simulink model "PILS"  (R2023a)
settings: Solver=daessc  StartTime=0.0  StopTime=1800  MaxStep=0.1  RelTol=1e-3
values from neighbouring files (symbols this model uses):
  Max_Power = 100000    [setHESSParam.m]    (also in setHESSParamv2.m)
  sim_case = i    [create_SOC_dataset.m]    (also in create_csv.m = 2; setHESSParam.m = 6; setHESSParamv2.m = 6)
undefined symbols (not defined in the file or in its folder): Battery, Capacitor, Ri
libraries: fl_lib x41, nesl_utility x22, dspstat3 x4, rllib x3, batteryecm_lib x1, autolibshared x1
(part 2 of 2)

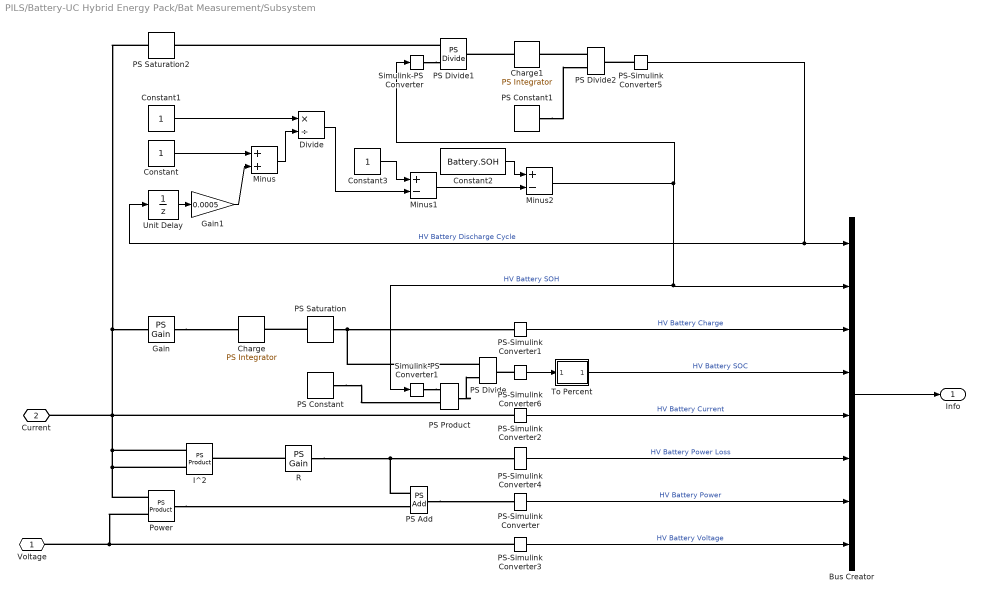
== system PILS/Battery-UC Hybrid Energy Pack/Bat Measurement/Subsystem ==
  Bus Creator : BusCreator  Inputs=8
  Charge : fl_lib/Physical Signals/Linear Operators/PS Integrator  reset_method=foundation.enum.IntegratorResetSpec.None  initial_condition_spec=foundation.enum.IntegratorICSpec.Internal  saturation_spec=foundation.enum.IntegratorSaturationSpec.None  saturation_source_spec=foundation.enum.IntegratorSaturationSourceSpec.Internal  x0=Battery.InitialCharge A*hr  xu=inf s  xl=-inf s
      settings: AttributesFormatString=%<x0> [%<x0_unit>]
  Charge1 : fl_lib/Physical Signals/Linear Operators/PS Integrator  reset_method=foundation.enum.IntegratorResetSpec.None  initial_condition_spec=foundation.enum.IntegratorICSpec.Internal  saturation_spec=foundation.enum.IntegratorSaturationSpec.None  saturation_source_spec=foundation.enum.IntegratorSaturationSourceSpec.Internal  x0=0 A*hr  xu=inf s  xl=-inf s
      settings: AttributesFormatString=%<x0> [%<x0_unit>]
  Constant : Constant
  Constant1 : Constant
  Constant2 : Constant  Value=Battery.SOH
  Constant3 : Constant
  Divide : Product  Inputs=*/
  Gain : fl_lib/Physical Signals/Functions/PS Gain  gain=-1
      settings: AttributesFormatString=%<gain>
  Gain1 : Gain  Gain=0.0005
  I^2 : fl_lib/Physical Signals/Functions/PS Product
  Minus : Sum
  Minus1 : Sum  Inputs=+-
  Minus2 : Sum  Inputs=+-
  PS Add : fl_lib/Physical Signals/Functions/PS Add
  PS Constant : fl_lib/Physical Signals/Sources/PS Constant  constant=Battery.Capacity A*hr
      settings: AttributesFormatString=%<constant> [%<constant_unit>]
  PS Constant1 : fl_lib/Physical Signals/Sources/PS Constant  constant=Battery.Capacity A*hr
  PS Divide : fl_lib/Physical Signals/Functions/PS Divide
  PS Divide1 : fl_lib/Physical Signals/Functions/PS Divide
  PS Divide2 : fl_lib/Physical Signals/Functions/PS Divide
  PS Product : fl_lib/Physical Signals/Functions/PS Product
  PS Saturation : fl_lib/Physical Signals/Nonlinear Operators/PS Saturation  upper_limit=Battery.Capacity A*hr  lower_limit=0 A*hr
      settings: AttributesFormatString=|
      | Upper: %<upper_limit>
      | Lower: %<lower_limit>
  PS Saturation2 : fl_lib/Physical Signals/Nonlinear Operators/PS Saturation  upper_limit=500 A  lower_limit=0 A
  PS-Simulink Converter : nesl_utility/PS-Simulink Converter  PhysicalDomain=network_engine_domain  SubClassName=ps_output  LeftPortType=input  RightPortType=output  PseudoPeriodic=off  Frequencies=[]  VectorFormat=1-D array  Unit=W  AffineConversion=off
  PS-Simulink Converter1 : nesl_utility/PS-Simulink Converter  PhysicalDomain=network_engine_domain  SubClassName=ps_output  LeftPortType=input  RightPortType=output  PseudoPeriodic=off  Frequencies=[]  VectorFormat=1-D array  Unit=A*hr  AffineConversion=off
  PS-Simulink Converter2 : nesl_utility/PS-Simulink Converter  PhysicalDomain=network_engine_domain  SubClassName=ps_output  LeftPortType=input  RightPortType=output  PseudoPeriodic=off  Frequencies=[]  VectorFormat=1-D array  Unit=A  AffineConversion=off
  PS-Simulink Converter3 : nesl_utility/PS-Simulink Converter  PhysicalDomain=network_engine_domain  SubClassName=ps_output  LeftPortType=input  RightPortType=output  PseudoPeriodic=off  Frequencies=[]  VectorFormat=1-D array  Unit=V  AffineConversion=off
  PS-Simulink Converter4 : nesl_utility/PS-Simulink Converter  PhysicalDomain=network_engine_domain  SubClassName=ps_output  LeftPortType=input  RightPortType=output  PseudoPeriodic=off  Frequencies=[]  VectorFormat=1-D array  Unit=W  AffineConversion=off
  PS-Simulink Converter5 : nesl_utility/PS-Simulink Converter  PhysicalDomain=network_engine_domain  SubClassName=ps_output  LeftPortType=input  RightPortType=output  PseudoPeriodic=off  Frequencies=[]  VectorFormat=inherit  Unit=1  AffineConversion=off
  PS-Simulink Converter6 : nesl_utility/PS-Simulink Converter  PhysicalDomain=network_engine_domain  SubClassName=ps_output  LeftPortType=input  RightPortType=output  PseudoPeriodic=off  Frequencies=[]  VectorFormat=1-D array  Unit=1  AffineConversion=off
  Power : fl_lib/Physical Signals/Functions/PS Product
  R : fl_lib/Physical Signals/Functions/PS Gain  gain=Battery.InternalResistance Ohm
      settings: AttributesFormatString=%<gain> [%<gain_unit>]
  Simulink-PS Converter : nesl_utility/Simulink-PS Converter  PhysicalDomain=network_engine_domain  SubClassName=ps_input  LeftPortType=input  RightPortType=output  PseudoPeriodic=off  Frequencies=[]  NoiseDistribution=none  NoiseParameters=[]  Unit=1  AffineConversion=off  FilteringAndDerivatives=provide  SimscapeFilterOrder=1  InputFilterTimeConstant=0.001  UdotUserProvided=0
  Simulink-PS Converter1 : nesl_utility/Simulink-PS Converter  PhysicalDomain=network_engine_domain  SubClassName=ps_input  LeftPortType=input  RightPortType=output  PseudoPeriodic=off  Frequencies=[]  NoiseDistribution=none  NoiseParameters=[]  Unit=1  AffineConversion=off  FilteringAndDerivatives=provide  SimscapeFilterOrder=1  InputFilterTimeConstant=0.001  UdotUserProvided=0
  To Percent : Subsystem
  Unit Delay : UnitDelay  SampleTime=-1  HasFrameUpgradeWarning=on
  Voltage : PMIOPort  Side=Left
  Current : PMIOPort  Port=2  Side=Left
  Info : Outport
  wires:
  PS-Simulink Converter4/1 -> Bus Creator/6  "HV Battery Power Loss"
  PS-Simulink Converter3/1 -> Bus Creator/8  "HV Battery Voltage"
  PS-Simulink Converter1/1 -> Bus Creator/3  "HV Battery Charge"
  Bus Creator/1 -> Info/1
  To Percent/1(Out1) -> Bus Creator/4  "HV Battery SOC"
  PS-Simulink Converter/1 -> Bus Creator/7  "HV Battery Power"
  PS-Simulink Converter6/1 -> To Percent/1(In1)
  PS-Simulink Converter2/1 -> Bus Creator/5  "HV Battery Current"
  Constant/1 -> Minus/1
  Gain1/1 -> Minus/2
  Unit Delay/1 -> Gain1/1
  Divide/1 -> Minus1/2
  Constant1/1 -> Divide/1
  Minus/1 -> Divide/2
  PS-Simulink Converter5/1 -> Bus Creator/1, Unit Delay/1  "HV Battery Discharge Cycle"
  Constant3/1 -> Minus1/1
  Constant2/1 -> Minus2/1
  Minus1/1 -> Minus2/2
  Minus2/1 -> Simulink-PS Converter1/1, Bus Creator/2, Simulink-PS Converter/1  "HV Battery SOH"
  connections:
  PS Divide/LConn1 -- PS-Simulink Converter1/LConn1 -- PS Saturation/RConn1
  Power/LConn1 -- Voltage/RConn1 -- PS-Simulink Converter3/LConn1
  R/RConn1 -- PS Add/LConn1 -- PS-Simulink Converter4/LConn1
  Power/LConn2 -- I^2/LConn1 -- Current/RConn1 -- PS Saturation2/LConn1 -- Gain/LConn1 -- PS-Simulink Converter2/LConn1 -- I^2/LConn2
  PS Add/RConn1 -- PS-Simulink Converter/LConn1
  R/LConn1 -- I^2/RConn1
  PS Saturation/LConn1 -- Charge/RConn1
  Gain/RConn1 -- Charge/LConn1
  PS-Simulink Converter6/LConn1 -- PS Divide/RConn1
  Power/RConn1 -- PS Add/LConn2
  PS Divide1/LConn1 -- PS Saturation2/RConn1
  Charge1/LConn1 -- PS Divide1/RConn1
  PS Divide2/LConn1 -- Charge1/RConn1
  PS Constant1/RConn1 -- PS Divide2/LConn2
  PS-Simulink Converter5/LConn1 -- PS Divide2/RConn1
  Simulink-PS Converter/RConn1 -- PS Divide1/LConn2
  PS Product/RConn1 -- PS Divide/LConn2
  PS Constant/RConn1 -- PS Product/LConn2
  Simulink-PS Converter1/RConn1 -- PS Product/LConn1

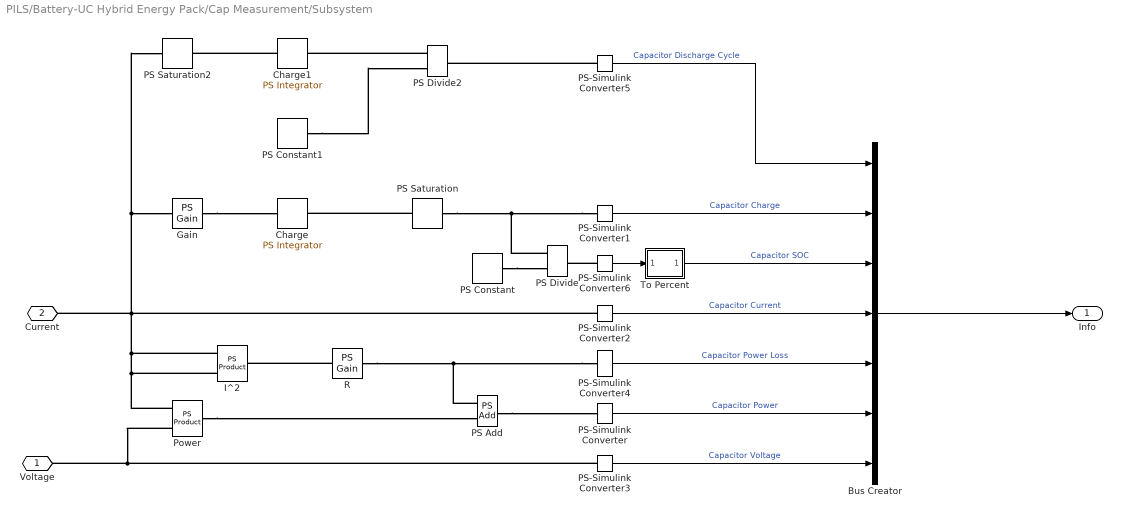
== system PILS/Battery-UC Hybrid Energy Pack/Cap Measurement/Subsystem ==
  Bus Creator : BusCreator  Inputs=7
  Charge : fl_lib/Physical Signals/Linear Operators/PS Integrator  reset_method=foundation.enum.IntegratorResetSpec.None  initial_condition_spec=foundation.enum.IntegratorICSpec.Internal  saturation_spec=foundation.enum.IntegratorSaturationSpec.None  saturation_source_spec=foundation.enum.IntegratorSaturationSourceSpec.Internal  x0=Capacitor.Capacity A*hr  xu=inf s  xl=-inf s
      settings: AttributesFormatString=%<x0> [%<x0_unit>]
  Charge1 : fl_lib/Physical Signals/Linear Operators/PS Integrator  reset_method=foundation.enum.IntegratorResetSpec.None  initial_condition_spec=foundation.enum.IntegratorICSpec.Internal  saturation_spec=foundation.enum.IntegratorSaturationSpec.None  saturation_source_spec=foundation.enum.IntegratorSaturationSourceSpec.Internal  x0=0 A*hr  xu=inf s  xl=-inf s
      settings: AttributesFormatString=%<x0> [%<x0_unit>]
  Gain : fl_lib/Physical Signals/Functions/PS Gain  gain=-1
      settings: AttributesFormatString=%<gain>
  I^2 : fl_lib/Physical Signals/Functions/PS Product
  PS Add : fl_lib/Physical Signals/Functions/PS Add
  PS Constant : fl_lib/Physical Signals/Sources/PS Constant  constant=Capacitor.Capacity A*hr
      settings: AttributesFormatString=%<constant> [%<constant_unit>]
  PS Constant1 : fl_lib/Physical Signals/Sources/PS Constant  constant=Capacitor.Capacity A*hr
      settings: AttributesFormatString=%<constant> [%<constant_unit>]
  PS Divide : fl_lib/Physical Signals/Functions/PS Divide
  PS Divide2 : fl_lib/Physical Signals/Functions/PS Divide
  PS Saturation : fl_lib/Physical Signals/Nonlinear Operators/PS Saturation  upper_limit=Capacitor.Capacity A*hr  lower_limit=0 A*hr
      settings: AttributesFormatString=|
      | Upper: %<upper_limit>
      | Lower: %<lower_limit>
  PS Saturation2 : fl_lib/Physical Signals/Nonlinear Operators/PS Saturation  upper_limit=500 A  lower_limit=0 A
  PS-Simulink Converter : nesl_utility/PS-Simulink Converter  PhysicalDomain=network_engine_domain  SubClassName=ps_output  LeftPortType=input  RightPortType=output  PseudoPeriodic=off  Frequencies=[]  VectorFormat=1-D array  Unit=W  AffineConversion=off
  PS-Simulink Converter1 : nesl_utility/PS-Simulink Converter  PhysicalDomain=network_engine_domain  SubClassName=ps_output  LeftPortType=input  RightPortType=output  PseudoPeriodic=off  Frequencies=[]  VectorFormat=1-D array  Unit=A*hr  AffineConversion=off
  PS-Simulink Converter2 : nesl_utility/PS-Simulink Converter  PhysicalDomain=network_engine_domain  SubClassName=ps_output  LeftPortType=input  RightPortType=output  PseudoPeriodic=off  Frequencies=[]  VectorFormat=1-D array  Unit=A  AffineConversion=off
  PS-Simulink Converter3 : nesl_utility/PS-Simulink Converter  PhysicalDomain=network_engine_domain  SubClassName=ps_output  LeftPortType=input  RightPortType=output  PseudoPeriodic=off  Frequencies=[]  VectorFormat=1-D array  Unit=V  AffineConversion=off
  PS-Simulink Converter4 : nesl_utility/PS-Simulink Converter  PhysicalDomain=network_engine_domain  SubClassName=ps_output  LeftPortType=input  RightPortType=output  PseudoPeriodic=off  Frequencies=[]  VectorFormat=1-D array  Unit=W  AffineConversion=off
  PS-Simulink Converter5 : nesl_utility/PS-Simulink Converter  PhysicalDomain=network_engine_domain  SubClassName=ps_output  LeftPortType=input  RightPortType=output  PseudoPeriodic=off  Frequencies=[]  VectorFormat=inherit  Unit=1  AffineConversion=off
  PS-Simulink Converter6 : nesl_utility/PS-Simulink Converter  PhysicalDomain=network_engine_domain  SubClassName=ps_output  LeftPortType=input  RightPortType=output  PseudoPeriodic=off  Frequencies=[]  VectorFormat=1-D array  Unit=1  AffineConversion=off
  Power : fl_lib/Physical Signals/Functions/PS Product
  R : fl_lib/Physical Signals/Functions/PS Gain  gain=Capacitor.InternalResistance Ohm
      settings: AttributesFormatString=%<gain> [%<gain_unit>]
  To Percent : Subsystem
  Voltage : PMIOPort  Side=Left
  Current : PMIOPort  Port=2  Side=Left
  Info : Outport
  wires:
  PS-Simulink Converter4/1 -> Bus Creator/5  "Capacitor Power Loss"
  PS-Simulink Converter3/1 -> Bus Creator/7  "Capacitor Voltage"
  PS-Simulink Converter1/1 -> Bus Creator/2  "Capacitor Charge"
  Bus Creator/1 -> Info/1
  To Percent/1(Out1) -> Bus Creator/3  "Capacitor SOC"
  PS-Simulink Converter/1 -> Bus Creator/6  "Capacitor Power"
  PS-Simulink Converter6/1 -> To Percent/1(In1)
  PS-Simulink Converter2/1 -> Bus Creator/4  "Capacitor Current"
  PS-Simulink Converter5/1 -> Bus Creator/1  "Capacitor Discharge Cycle"
  connections:
  PS-Simulink Converter1/LConn1 -- PS Divide/LConn1 -- PS Saturation/RConn1
  PS-Simulink Converter3/LConn1 -- Power/LConn1 -- Voltage/RConn1
  PS-Simulink Converter4/LConn1 -- R/RConn1 -- PS Add/LConn1
  Current/RConn1 -- PS Saturation2/LConn1 -- Gain/LConn1 -- PS-Simulink Converter2/LConn1 -- I^2/LConn2 -- I^2/LConn1 -- Power/LConn2
  PS Add/RConn1 -- PS-Simulink Converter/LConn1
  R/LConn1 -- I^2/RConn1
  PS Saturation/LConn1 -- Charge/RConn1
  Gain/RConn1 -- Charge/LConn1
  PS-Simulink Converter6/LConn1 -- PS Divide/RConn1
  Power/RConn1 -- PS Add/LConn2
  PS Constant/RConn1 -- PS Divide/LConn2
  Charge1/LConn1 -- PS Saturation2/RConn1
  PS-Simulink Converter5/LConn1 -- PS Divide2/RConn1
  PS Divide2/LConn1 -- Charge1/RConn1
  PS Constant1/RConn1 -- PS Divide2/LConn2

== system PILS/Battery-UC Hybrid Energy Pack/Bat Measurement/Subsystem/To Percent ==
  In1 : Inport
  Unit Conversion : UnitConversion
  Out1 : Outport  Unit=%
      settings: AttributesFormatString=%<Unit>
  wires:
  Unit Conversion/1 -> Out1/1
  In1/1 -> Unit Conversion/1

== system PILS/Battery-UC Hybrid Energy Pack/Cap Measurement/Subsystem/To Percent ==
  In1 : Inport
  Unit Conversion : UnitConversion
  Out1 : Outport  Unit=%
      settings: AttributesFormatString=%<Unit>
  wires:
  Unit Conversion/1 -> Out1/1
  In1/1 -> Unit Conversion/1

== matlab function PILS/RL-based EMS/SAC/MATLAB Function ==
  data: Pwr_Dmd input; Bat_Rate input; B_Rate output; Cap_Rate input; Cap_SOC input; C_Rate output; Cap_over_discharge output; Bat_over_discharge output; Cap_over_charge output; Bat_over_charge output; Bat_SOC input
function [B_Rate, C_Rate, Cap_over_discharge, Bat_over_discharge, Cap_over_charge, Bat_over_charge] = filter(Pwr_Dmd, Bat_Rate, Cap_Rate, Cap_SOC, Bat_SOC)

B_Rate = Bat_Rate;
C_Rate = Cap_Rate;

Bat_over_discharge = 0;
Bat_over_charge = 0;

Cap_over_discharge = 0;
Cap_over_charge = 0;

%{
if (Pwr_Dmd >= 0 && Cap_SOC <= 0.5)

    C_Rate = 0;
    Cap_over_discharge = Cap_Rate;

end

if (Pwr_Dmd >= 0 && Bat_SOC <= 0.2)

    B_Rate = 0;
    Bat_over_discharge = Bat_Rate;

end

if (Pwr_Dmd < 0 && Bat_SOC >= 1)

    B_Rate = 0;
    Bat_over_charge = Bat_Rate;

end

if (Pwr_Dmd < 0 && Cap_SOC >= 1)

    C_Rate = 0;
    Cap_over_charge = Cap_Rate;

end
%}

== matlab function PILS/RL-based EMS/REF/MATLAB Function1 ==
  data: isDone output; Bat_Pwr input; Cap_Pwr input; Pwr_Dmd input; Cap_SOC input; sim_case input; current_time input
function isDone = check(Bat_Pwr, Cap_Pwr, Pwr_Dmd, Cap_SOC, sim_case, current_time)


flag = 0;


if Cap_SOC < 0.2
    flag = 1;
end


if sim_case == 2
    if current_time > 1372
        flag = 1;
    end

elseif sim_case == 3
    if current_time > 1369
        flag = 1;
    end

elseif sim_case == 4
    if current_time > 1022
        flag = 1;
    end

elseif sim_case == 5
    if current_time > 1477
        flag = 1;
    end

elseif sim_case == 6
    if current_time > 1800
        flag = 1;
    end
end

isDone = flag;

== matlab function PILS/RL-based EMS/REF/MATLAB Function5 ==
  data: Cap_Voltage input; reward output; Cap_SOC input; Pwr_Dmd input; Pwr_Dmd_Derivative input; r1 output; r2 output; r3 output; r4 output; Total_Reward output; B_Rate input; C_Rate input
function [reward, r1, r2, r3, r4, Total_Reward] = cal_reward(Cap_Voltage, Cap_SOC, Pwr_Dmd, Pwr_Dmd_Derivative, B_Rate, C_Rate)

r1 = 0;
r2 = 0;
r3 = 0;
r4 = 0;


MAX = 100000;

w = Pwr_Dmd / MAX;

reward = Cap_SOC ^ 2;
reward = 0;

Bat_Pwr = Pwr_Dmd * B_Rate;
UC_Pwr = Pwr_Dmd * C_Rate;

if (Cap_SOC > 0.65) || (Cap_SOC > 0.65 && Pwr_Dmd < 0)
    r1 = (1 - ((MAX - UC_Pwr)/MAX)^0.4);
end

if (Cap_SOC < 0.65)
    r2 = 1 - ((MAX - Bat_Pwr)/MAX)^0.4;
end

if Cap_SOC < 0.65 && Pwr_Dmd > 0
    r3 = -(1-((MAX-UC_Pwr)/MAX)^0.4);
end

if Cap_Voltage > 600
    reward = -(Cap_SOC ^ 2);
    r1 = - (r1*10);
    r2 = - r2;
end

% Total_Reward = 0;
Total_Reward = reward + r1 + r2 + r3 + r4;

== matlab function PILS/RL-based EMS/Rule-based/MATLAB Function ==
  data: Pwr_Dmd input; Pwr_Dmd_Der input; Bat_Rate output; UC_SOC input; UC_Rate output
function [Bat_Rate, UC_Rate] = fcn(Pwr_Dmd, Pwr_Dmd_Der, UC_SOC)

if Pwr_Dmd < 0 % Regenerative Breaking

    if UC_SOC >= 1
        UC_Rate = 0;
        Bat_Rate = 1;
    else
        UC_Rate = 1;
        Bat_Rate = 0;
    end

else

    if UC_SOC <= 0.5
        UC_Rate = 0;
        Bat_Rate = 1;
    else

        if Pwr_Dmd_Der > 0

            % UC_Rate = 0.3;
            % Bat_Rate = 0.7;

            UC_Rate = 0.6;
            Bat_Rate = 0.4;




        elseif Pwr_Dmd_Der == 0
            UC_Rate = 0.3;
            Bat_Rate = 0.7;
        else
            UC_Rate = 0;
            Bat_Rate = 1;
        end
    end
end

== matlab function PILS/RL-based EMS/SAC/MATLAB Function2 ==
  data: Pwr_Dmd input; res output; Cap_SOC input; Bat_SOC input
function res = fcn(Pwr_Dmd, Cap_SOC, Bat_SOC)


Pwr_Dmd = sprintf('%.3f', Pwr_Dmd);
Cap_SOC = sprintf('%.3f', Cap_SOC);
Bat_SOC = sprintf('%.3f', Bat_SOC);

input = Pwr_Dmd + "," + Cap_SOC + "," + Bat_SOC;


%{ 



write(client, input, "string")

output = readline(client);output = str2double(output);

clear client

res = output;

%}

% res = test_function(Pwr_Dmd, Cap_SOC, Bat_SOC);

res = tcp_test(Pwr_Dmd, Cap_SOC, Bat_SOC);


% res = 0;

== matlab function PILS/RL-based EMS/SAC/MATLAB Function1 ==
  data: isDone output; Bat_Pwr input; Cap_Pwr input; Pwr_Dmd input; Cap_SOC input; sim_case input; current_time input
function isDone = check(Bat_Pwr, Cap_Pwr, Pwr_Dmd, Cap_SOC, sim_case, current_time)


flag = 0;


if Cap_SOC < 0.2
    flag = 1;
end


if sim_case == 2
    if current_time > 1372
        flag = 1;
    end

elseif sim_case == 3
    if current_time > 1369
        flag = 1;
    end

elseif sim_case == 4
    if current_time > 1022
        flag = 1;
    end

elseif sim_case == 5
    if current_time > 1477
        flag = 1;
    end

elseif sim_case == 6
    if current_time > 1800
        flag = 1;
    end
end

isDone = flag;

== matlab function PILS/RL-based EMS/SAC/MATLAB Function5 ==
  data: Cap_Voltage input; reward output; Cap_SOC input; Pwr_Dmd input; Pwr_Dmd_Derivative input; r1 output; r2 output; r3 output; r4 output; Total_Reward output; B_Rate input; C_Rate input; Bat_SOH input
function [reward, r1, r2, r3, r4, Total_Reward] = cal_reward(Cap_Voltage, Cap_SOC, Pwr_Dmd, Pwr_Dmd_Derivative, B_Rate, C_Rate, Bat_SOH)

r1 = 0;
r2 = 0;
r3 = 0;
r4 = 0;

MAX = 100000;

w = Pwr_Dmd / MAX;

tmp = 1 - Bat_SOH;
Bat_SOH = 1 - (10000 * tmp);

reward = Cap_SOC + Bat_SOH;

% Discharge Reward
if (Cap_SOC > 0.55 && Pwr_Dmd > 0) && (Pwr_Dmd_Derivative > 0)
    r1 = w * C_Rate;
end

% Charge Reward
if (Cap_SOC < 1 && Pwr_Dmd < 0)
    r2 = C_Rate;
end

% Overdischarge Penalty
if Cap_SOC < 0.55 && Pwr_Dmd > 0
    r3 = -(C_Rate);
    reward = - (Cap_SOC + Bat_SOH);
end

% Overcharge Penalty
if Cap_Voltage > 600 && Pwr_Dmd < 0
    r4 = -(C_Rate);
    reward = - (Cap_SOC + Bat_SOH);
end

% Overcharge Penalty
if Cap_Voltage > 600
    r1 = -r1;
    r2 = -r2;
    reward = - (Cap_SOC + Bat_SOH);
end

Total_Reward = reward + r1 + r2 + r3 + r4;

== matlab function PILS/RL-based EMS/DQN/MATLAB Function ==
  data: Pwr_Dmd input; Bat_Rate input; B_Rate output; Cap_Rate input; Cap_SOC input; C_Rate output; Cap_over_discharge output; Bat_over_discharge output; Cap_over_charge output; Bat_over_charge output; Bat_SOC input
function [B_Rate, C_Rate, Cap_over_discharge, Bat_over_discharge, Cap_over_charge, Bat_over_charge] = filter(Pwr_Dmd, Bat_Rate, Cap_Rate, Cap_SOC, Bat_SOC)

B_Rate = Bat_Rate;
C_Rate = Cap_Rate;

Bat_over_discharge = 0;
Bat_over_charge = 0;

Cap_over_discharge = 0;
Cap_over_charge = 0;

%{
if (Pwr_Dmd >= 0 && Cap_SOC <= 0.5)

    C_Rate = 0;
    Cap_over_discharge = Cap_Rate;

end

if (Pwr_Dmd >= 0 && Bat_SOC <= 0.2)

    B_Rate = 0;
    Bat_over_discharge = Bat_Rate;

end

if (Pwr_Dmd < 0 && Bat_SOC >= 1)

    B_Rate = 0;
    Bat_over_charge = Bat_Rate;

end

if (Pwr_Dmd < 0 && Cap_SOC >= 1)

    C_Rate = 0;
    Cap_over_charge = Cap_Rate;

end
%}

== matlab function PILS/RL-based EMS/DQN/MATLAB Function1 ==
  data: isDone output; Bat_Pwr input; Cap_Pwr input; Pwr_Dmd input; Cap_SOC input; sim_case input; current_time input
function isDone = check(Bat_Pwr, Cap_Pwr, Pwr_Dmd, Cap_SOC, sim_case, current_time)


flag = 0;


if Cap_SOC < 0.2
    flag = 1;
end


if sim_case == 2
    if current_time > 1372
        flag = 1;
    end

elseif sim_case == 3
    if current_time > 1369
        flag = 1;
    end

elseif sim_case == 4
    if current_time > 1022
        flag = 1;
    end

elseif sim_case == 5
    if current_time > 1477
        flag = 1;
    end

elseif sim_case == 6
    if current_time > 1800
        flag = 1;
    end
end

isDone = flag;

== matlab function PILS/RL-based EMS/DQN/MATLAB Function5 ==
  data: Bat_SOC input; reward output; Cap_SOC input; Pwr_Dmd input; Pwr_Dmd_Derivative input; r1 output; r2 output; r3 output; r4 output; Total_Reward output; B_Rate input; C_Rate input
function [reward, r1, r2, r3, r4, Total_Reward] = cal_reward(Bat_SOC, Cap_SOC, Pwr_Dmd, Pwr_Dmd_Derivative, B_Rate, C_Rate)

r1 = 0;
r2 = 0;
r3 = 0;
r4 = 0;

w = Pwr_Dmd / 100000;

reward = Cap_SOC;

% Discharge Reward
if (Cap_SOC > 0.65 && Pwr_Dmd > 0) && (Pwr_Dmd_Derivative > 0)
    r1 = w * C_Rate;
end

% Charge Reward
if (Cap_SOC < 1 && Pwr_Dmd < 0)
    r2 = C_Rate;
end

% Overdischarge Penalty
if Cap_SOC < 0.65 && Pwr_Dmd > 0
    r3 = -2 * (C_Rate);
end

% Overcharge Penalty
if Cap_SOC >= 1 && Pwr_Dmd < 0
    r4 = -2 * (C_Rate);
end

Total_Reward = reward + r1 + r2 + r3 + r4;

== matlab function PILS/RL-based EMS/DQN/MATLAB Function2 ==
  data: Action input; bat_rate output; cap_rate output
function [bat_rate, cap_rate]= fcn(Action)

% Action means cap rate (1 ~ 11)
flag = Action - 1; % (0, 1, 2, 3, 4, 5, 6, 7, 8, 9, 10)

cap_rate = flag * 0.1;
bat_rate = 1 - cap_rate;

== matlab function PILS/RL-based EMS/REF/MATLAB Function ==
  data: Pwr_Dmd input; Bat_Rate input; B_Rate output; Cap_Rate input; Cap_SOC input; C_Rate output; Cap_over_discharge output; Bat_over_discharge output; Cap_over_charge output; Bat_over_charge output; Bat_SOC input
function [B_Rate, C_Rate, Cap_over_discharge, Bat_over_discharge, Cap_over_charge, Bat_over_charge] = filter(Pwr_Dmd, Bat_Rate, Cap_Rate, Cap_SOC, Bat_SOC)

B_Rate = Bat_Rate;
C_Rate = Cap_Rate;

Bat_over_discharge = 0;
Bat_over_charge = 0;

Cap_over_discharge = 0;
Cap_over_charge = 0;

%{
if (Pwr_Dmd >= 0 && Cap_SOC <= 0.5)

    C_Rate = 0;
    Cap_over_discharge = Cap_Rate;

end

if (Pwr_Dmd >= 0 && Bat_SOC <= 0.2)

    B_Rate = 0;
    Bat_over_discharge = Bat_Rate;

end

if (Pwr_Dmd < 0 && Bat_SOC >= 1)

    B_Rate = 0;
    Bat_over_charge = Bat_Rate;

end

if (Pwr_Dmd < 0 && Cap_SOC >= 1)

    C_Rate = 0;
    Cap_over_charge = Cap_Rate;

end
%}
